simulink model "GonzalezGC21210380"  (R2024b)
settings: Solver=ode15s  StartTime=0.0  StopTime=30  MaxStep=1E-3  RelTol=1e-3
libraries: slpidlib x1
settings DataIOCC: ReturnWorkspaceOutputs=off  TimeSaveName=t
settings DebuggingCC: AlgebraicLoopMsg=none  ArtificialAlgebraicLoopMsg=none  MaxConsecutiveZCsMsg=none  OperatingPointInterfaceChecksumMismatchMsg=none

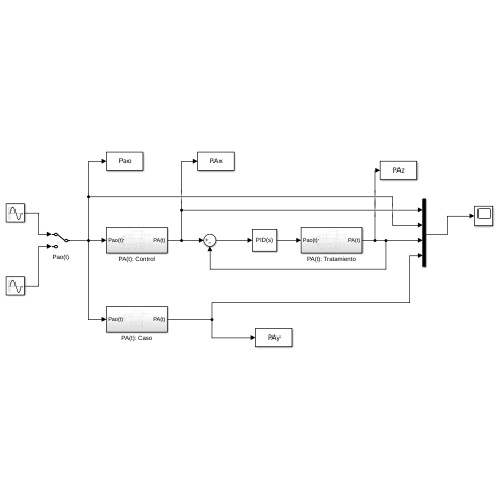
[thumbnail: Simulink's stored preview of the top-level diagram]
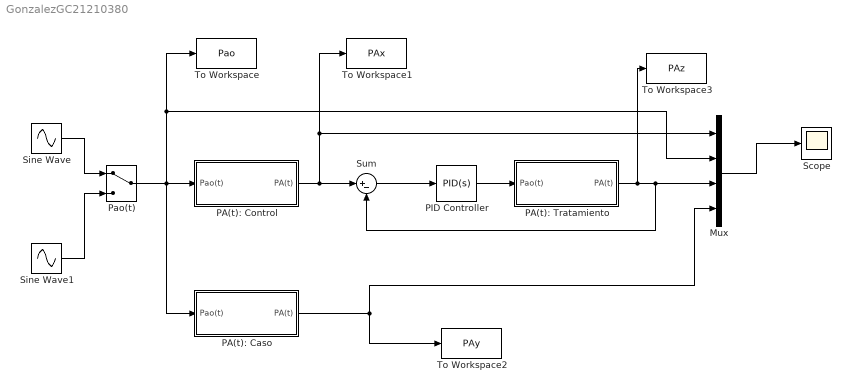
== system GonzalezGC21210380 ==
  Mux : Mux
  PA(t): Caso : Subsystem
  PA(t): Control : Subsystem
  PA(t): Tratamiento : Subsystem
  PID Controller : slpidlib/PID Controller  Controller=PID  Form=Parallel  TimeDomain=Continuous-time  UseExternalTs=off  SampleTime=-1  IntegratorMethod=Forward Euler  FilterMethod=Forward Euler  ControllerParametersSource=internal  P=15.8954  I=452.1208  UseKiTs=off  D=0.042897  UseExternalDerivativeSource=off  N=198.6514  UseFilter=on  TunerSelectOption=Transfer Function Based (PID Tuner App)  InitialConditionSource=internal  InitialConditionForIntegrator=0  InitialConditionForFilter=0  DifferentiatorICPrevScaledInput=0  ExternalReset=none  TrackingMode=off  Kt=1  LimitOutput=off  SatLimitsSource=internal  UpperSaturationLimit=inf  LowerSaturationLimit=-inf  LinearizeAsGain=on  AntiWindupMode=none  Kb=1  LimitIntegrator=off  UpperIntegratorSaturationLimit=inf  LowerIntegratorSaturationLimit=-inf  POutMin=[]  POutMax=[]  IOutMin=[]  IOutMax=[]  DOutMin=[]  DOutMax=[]  NOutMin=[]  NOutMax=[]  SumOutMin=[]  SumOutMax=[]  SaturationOutMin=[]  SaturationOutMax=[]  PParamMin=[]  PParamMax=[]  IParamMin=[]  IParamMax=[]  DParamMin=[]  DParamMax=[]  NParamMin=[]  NParamMax=[]  KbParamMin=[]  KbParamMax=[]  KtParamMin=[]  KtParamMax=[]  KbOutMin=[]  KbOutMax=[]  KtOutMin=[]  KtOutMax=[]  IntegratorOutMin=[]  IntegratorOutMax=[]  FilterOutMin=[]  FilterOutMax=[]  SumI1OutMin=[]  SumI1OutMax=[]  SumI2OutMin=[]  SumI2OutMax=[]  SumI3OutMin=[]  SumI3OutMax=[]  SumI4OutMin=[]  SumI4OutMax=[]  SumDOutMin=[]  SumDOutMax=[]  DifferentiatorOutMin=[]  DifferentiatorOutMax=[]  FilterDiffOutCoefMin=[]  FilterDiffOutCoefMax=[]  ReciprocalOutMin=[]  ReciprocalOutMax=[]  SumDenOutMin=[]  SumDenOutMax=[]  SumNumOutMin=[]  SumNumOutMax=[]  DivideOutMin=[]  DivideOutMax=[]  UdiffTsProdOutMin=[]  UdiffTsProdOutMax=[]  NTsProdOutMin=[]  NTsProdOutMax=[]  UintegralTsProdOutMin=[]  UintegralTsProdOutMax=[]  UngainTsProdOutMin=[]  UngainTsProdOutMax=[]  ClampingZeroOutDataTypeStr=Inherit: Inherit via back propagation  ClampingZeroOutMin=[]  ClampingZeroOutMax=[]  FilterDenConstantOutDataTypeStr=Inherit: Inherit via back propagation  FilterDenConstantOutMin=[]  FilterDenConstantOutMax=[]  PCopyOutDataTypeStr=Inherit: Inherit via back propagation  PCopyOutMin=[]  PCopyOutMax=[]  NCopyOutDataTypeStr=Inherit: Inherit via back propagation  NCopyOutMin=[]  NCopyOutMax=[]  IntegratorContinuousStateAttributes=''  IntegratorStateMustResolveToSignalObject=off  IntegratorRTWStateStorageClass=Auto  FilterContinuousStateAttributes=''  FilterStateMustResolveToSignalObject=off  FilterRTWStateStorageClass=Auto  ParallelPVariant=InternalParameters  IdealPVariant=Disabled  IVariant=InternalParameters  DVariant=InternalParameters  IntegratorVariant=Continuous  SatVariant=Disabled  AWVariant=Passthrough  PCopyVariant=Disabled  TRVariant=Disabled  FdbkBlocksVariant=Forward  IdealPFdbkVariant=Disabled  SatFdbkVariant=Disabled  DerivativeFilterVariant=ContFilter  NVariant=InternalParameters  NCopyVariant=Disabled  FilterICVariant=InternalICsFilter  IntegratorICVariant=InternalICs  ExternalResetVariant=Disabled  TRSumVariant=Passthrough  SumFdbkVariant=Disabled  SumVariant=Sum_PID  TsampFilterVariant=InternalTs  TsampNgainVariant=Passthrough  TsampIntegralVariant=Disabled_SignalSpec  ExternalSaturationOutDataTypeStr=Inherit: Same as second input  DerivativeSourceVariant=ErrorSignal  PreIntVariant=InternalPreInt
  Pao(t) : ManualSwitch
  Scope : Scope
  Sine Wave : Sin  Amplitude=2.5  Frequency=pi/2  SampleTime=0
  Sine Wave1 : Sin  Amplitude=1.5  Frequency=pi  SampleTime=0
  Sum : Sum  Inputs=|+-
  To Workspace : ToWorkspace  VariableName=Pao  SampleTime=-1
  To Workspace1 : ToWorkspace  VariableName=PAx  SampleTime=-1
  To Workspace2 : ToWorkspace  VariableName=PAy  SampleTime=-1
  To Workspace3 : ToWorkspace  VariableName=PAz  SampleTime=-1
  wires:
  Sine Wave1/1 -> Pao(t)/2
  Pao(t)/1 -> PA(t): Caso/1(Pao(t)), To Workspace/1, Mux/2, PA(t): Control/1(Pao(t))
  PA(t): Control/1(PA(t)) -> To Workspace1/1, Mux/1, Sum/1
  Sum/1 -> PID Controller/1
  Mux/1 -> Scope/1
  PA(t): Caso/1(PA(t)) -> To Workspace2/1, Mux/4
  PA(t): Tratamiento/1(PA(t)) -> To Workspace3/1, Mux/3, Sum/2
  PID Controller/1 -> PA(t): Tratamiento/1(Pao(t))
  Sine Wave/1 -> Pao(t)/1

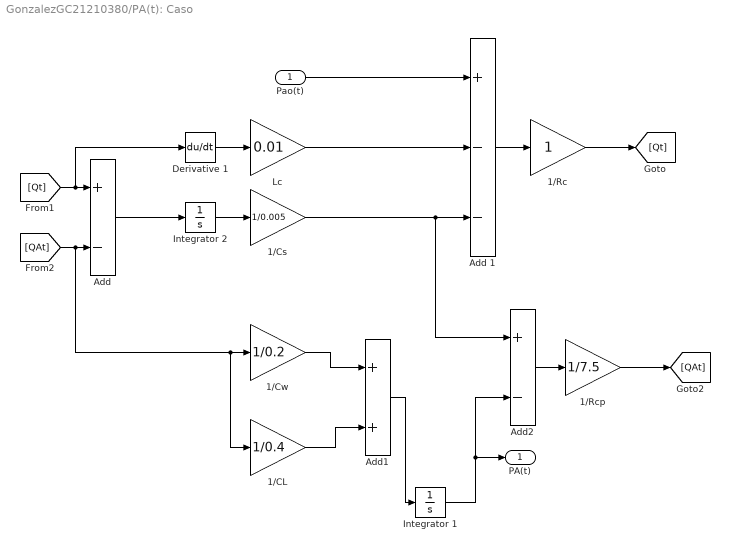
== system GonzalezGC21210380/PA(t): Caso ==
  Pao(t) : Inport
  1/CL : Gain  Gain=1/0.4
  1/Cs : Gain  Gain=1/0.005
  1/Cw : Gain  Gain=1/0.2
  1/Rc : Gain
  1/Rcp : Gain  Gain=1/7.5
  Add : Sum  Inputs=+-
  Add 1 : Sum  Inputs=+--
  Add1 : Sum
  Add2 : Sum  Inputs=+-
  Derivative 1 : Derivative
  Integrator 1 : Integrator
  Integrator 2 : Integrator
  Lc : Gain  Gain=0.01
  PA(t) : Outport
  wires:
  Add/1 -> Integrator 2/1
  Integrator 2/1 -> 1/Cs/1
  [QAt] -> 1/CL/1, 1/Cw/1, Add/2
  1/Cw/1 -> Add1/1
  Add1/1 -> Integrator 1/1
  1/CL/1 -> Add1/2
  [Qt] -> Derivative 1/1, Add/1
  Add 1/1 -> 1/Rc/1
  1/Cs/1 -> Add2/1, Add 1/3
  Add2/1 -> 1/Rcp/1
  1/Rcp/1 -> [QAt]
  Lc/1 -> Add 1/2
  Pao(t)/1 -> Add 1/1
  Derivative 1/1 -> Lc/1
  1/Rc/1 -> [Qt]
  Integrator 1/1 -> PA(t)/1, Add2/2

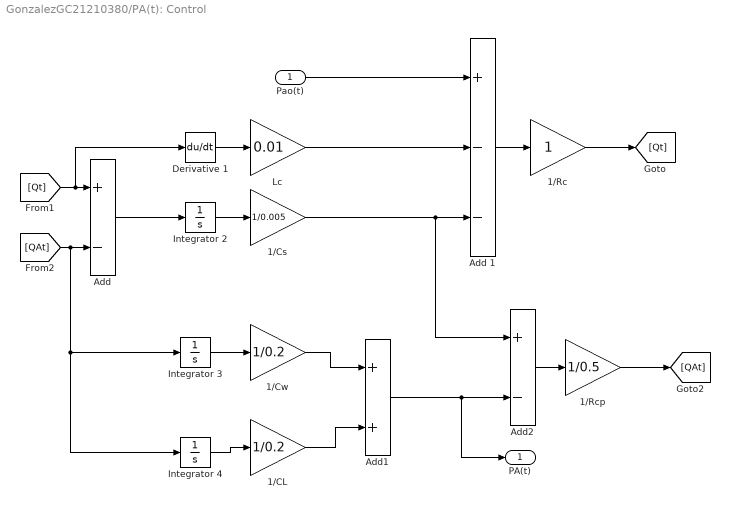
== system GonzalezGC21210380/PA(t): Control ==
  Pao(t) : Inport
  1/CL : Gain  Gain=1/0.2
  1/Cs : Gain  Gain=1/0.005
  1/Cw : Gain  Gain=1/0.2
  1/Rc : Gain
  1/Rcp : Gain  Gain=1/0.5
  Add : Sum  Inputs=+-
  Add 1 : Sum  Inputs=+--
  Add1 : Sum
  Add2 : Sum  Inputs=+-
  Derivative 1 : Derivative
  Integrator 2 : Integrator
  Integrator 3 : Integrator
  Integrator 4 : Integrator
  Lc : Gain  Gain=0.01
  PA(t) : Outport
  wires:
  Pao(t)/1 -> Add 1/1
  Lc/1 -> Add 1/2
  Derivative 1/1 -> Lc/1
  Integrator 2/1 -> 1/Cs/1
  Add 1/1 -> 1/Rc/1
  [Qt] -> Derivative 1/1, Add/1
  [QAt] -> Integrator 4/1, Integrator 3/1, Add/2
  Add/1 -> Integrator 2/1
  1/Rc/1 -> [Qt]
  1/Cw/1 -> Add1/1
  1/CL/1 -> Add1/2
  Integrator 3/1 -> 1/Cw/1
  Integrator 4/1 -> 1/CL/1
  Add1/1 -> PA(t)/1, Add2/2
  1/Cs/1 -> Add2/1, Add 1/3
  Add2/1 -> 1/Rcp/1
  1/Rcp/1 -> [QAt]

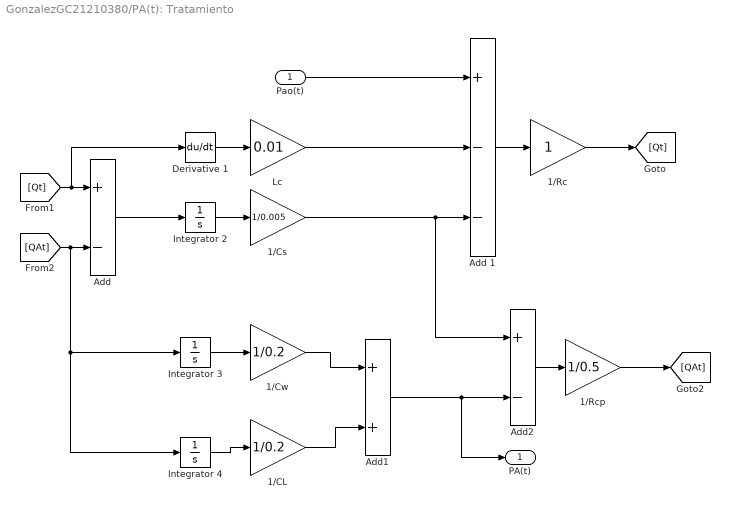
== system GonzalezGC21210380/PA(t): Tratamiento ==
  Pao(t) : Inport
  1/CL : Gain  Gain=1/0.2
  1/Cs : Gain  Gain=1/0.005
  1/Cw : Gain  Gain=1/0.2
  1/Rc : Gain
  1/Rcp : Gain  Gain=1/0.5
  Add : Sum  Inputs=+-
  Add 1 : Sum  Inputs=+--
  Add1 : Sum
  Add2 : Sum  Inputs=+-
  Derivative 1 : Derivative
  Integrator 2 : Integrator
  Integrator 3 : Integrator
  Integrator 4 : Integrator
  Lc : Gain  Gain=0.01
  PA(t) : Outport
  wires:
  Add/1 -> Integrator 2/1
  Integrator 2/1 -> 1/Cs/1
  [QAt] -> Integrator 4/1, Integrator 3/1, Add/2
  Integrator 4/1 -> 1/CL/1
  1/Cw/1 -> Add1/1
  Add1/1 -> PA(t)/1, Add2/2
  Integrator 3/1 -> 1/Cw/1
  1/CL/1 -> Add1/2
  [Qt] -> Derivative 1/1, Add/1
  Add 1/1 -> 1/Rc/1
  1/Cs/1 -> Add2/1, Add 1/3
  Add2/1 -> 1/Rcp/1
  1/Rcp/1 -> [QAt]
  Lc/1 -> Add 1/2
  Pao(t)/1 -> Add 1/1
  Derivative 1/1 -> Lc/1
  1/Rc/1 -> [Qt]
